simulink model "NavigationRocketPlant"  (R2025b)
settings: Solver=ode5  StartTime=0.0  StopTime=350  RelTol=1e-3
PostLoadFcn:
  | addpath('settings/')
  | addpath('settings/environment/')
  | 
  | run sensorSettings.m
InitFcn:
  | run(fullfile(fileparts(get_param(bdroot,'FileName')),'..','rocketPlantMain.m'))
undefined symbols (not defined in the file): Airbrake, AirbrakeInitialState, ba0, bg0, CdLookup, DiscIntNeverNeededParam, dspblkCoreblockFVToolHelper, Environment, gcbh, GNSSConfig, GNSSInitialState, LLA0, MEKF, p0, P0, pressure0, q0, Rocket, RocketInitialState, Sensor, stationaryTime, v0, Weather
libraries: simulink x2, dspmathops x1
(part 3 of 3)

== matlab function NavigationRocketPlant/Sensors/GNSS/GNSS_Receiver ==
  data: truth_NEU input; LLA_deg_m output; fix_info output; time_s input; reference input; state_in input Bus: GNSSReceiverStateBus; GNSSConfig parameter; state_out output Bus: GNSSReceiverStateBus
function [LLA_deg_m, fix_info, state_out] = GNSSReceiver( ...
    truth_NEU, time_s, reference, state_in, GNSSConfig)
% Position only: latitude [deg], longitude [deg], ellipsoid height [m].
% Acquisition error and metadata are delayed together; no velocity output.
% All noise streams, correlated errors and delayed packets are explicit.
% GNSS_State (Unit Delay) supplies the initialized state and stores updates.
state_out = state_in;
%GNSSPOSITIONSTEP Acquire, perturb and deliver a position-only GNSS fix.
%   truth_NEU = [north; east; absolute_altitude; vNorth; vEast; vUp], SI.
%   LLA_deg_m = [latitude_deg; longitude_deg; absolute_altitude_m]. The altitude
%   datum is inherited from the trajectory; no geoid correction is implied.
%   fix_info = [fresh; valid; acquisitionTime; age; sigmaN; sigmaE; sigmaD;
%           reasonCode]. Sigmas describe aggregate metric NED position noise.
%   reasonCode is a bit mask: 1 invalid truth, 2 startup/specified outage,
%   4 conservative receiver dynamics gate, 8 reacquisition, 16 packet loss,
%   32 stale. A received invalid-fix packet is fresh but invalid. A packet
%   loss notification is neither fresh nor valid, and never changes LLA.
%
%   Correlated residuals aggregate post-solution atmospheric/orbit/receiver
%   effects. Ground multipath and quality/outlier windows are configurable
%   scenarios, not satellite-geometry predictions. Velocity truth is used
%   only to check the receiver envelope; GNSS velocity is never produced.
%   Call gnssPositionInitialize to reset before each simulation.

    assert(isequal(size(truth_NEU), [6, 1]));
    assert(isfinite(time_s) && time_s >= 0.0);
    tolerance = 1.0e-9 * max(1.0, abs(time_s));
    assert(time_s >= state_out.previousStepTime - tolerance);
    state_out.previousStepTime = time_s;

    if time_s >= state_out.nextAcquisitionTime - tolerance
        % Receiver clock Ts/TransportSubsteps hits every acquisition epoch.
        % If a standalone caller skips ticks after a gap,
        % acquire the current truth once; do not invent historical fixes.
        state_out.nextAcquisitionTime = ...
            (floor((time_s + tolerance) / GNSSConfig.Ts) + 1.0) * GNSSConfig.Ts;
        [packetLLA, packetInfo, state_out] = acquirePosition( ...
            truth_NEU, time_s, reference, GNSSConfig, state_out);
        assert(state_out.queueCount < 32.0);
        tail = mod(state_out.queueHead + state_out.queueCount - 1.0, 32.0) + 1.0;
        state_out.queueLLA(:, tail) = packetLLA;
        state_out.queueInfo(:, tail) = packetInfo;
        state_out.queueDueTime(tail) = time_s + GNSSConfig.Delay;
        state_out.queueCount = state_out.queueCount + 1.0;
    end

    fresh = 0.0;
    % Fixed-size loop is compatible with generated MATLAB Function code.
    for packet = 1:32
        if state_out.queueCount <= 0.0
            break;
        end
        head = state_out.queueHead;
        if state_out.queueDueTime(head) > time_s + tolerance
            break;
        end
        arrived = state_out.queueInfo(:, head);
        if arrived(2) > 0.5
            state_out.heldLLA = state_out.queueLLA(:, head);
        end
        state_out.heldInfo = arrived;
        fresh = max(fresh, arrived(1));
        state_out.queueDueTime(head) = realmax;
        state_out.queueHead = mod(head, 32.0) + 1.0;
        state_out.queueCount = state_out.queueCount - 1.0;
    end

    LLA_deg_m = state_out.heldLLA;
    fix_info = state_out.heldInfo;
    fix_info(1) = fresh;
    fix_info(4) = max(0.0, time_s - fix_info(3));
    if fix_info(4) > GNSSConfig.MaxAge + tolerance
        fix_info(2) = 0.0;
        if mod(floor(fix_info(8) / 32.0), 2.0) == 0.0
            fix_info(8) = fix_info(8) + 32.0;
        end
    end
% Hold the delivered-packet marker across the asynchronous rate transfer.
% GNSS_Consume produces the single fresh pulse at the IMU polling tick.
fix_info(1) = state_out.heldInfo(1);
LLA_deg_m(3) = LLA_deg_m(3) + GNSSConfig.GeoidSeparation;
end

function [lla, info, state] = acquirePosition( ...
    truthNEU6, time_s, referenceLLArad, cfg, state)
    white = zeros(3, 1);
    phiSlow = exp(-cfg.Ts / cfg.Correlated.Tau);
    phiMultipath = exp(-cfg.Ts / cfg.Multipath.Tau);
    for axis = 1:3
        [normalWhite, state.rng(axis)] = normalDraw(state.rng(axis));
        [normalSlow, state.rng(axis + 3)] = ...
            normalDraw(state.rng(axis + 3));
        [normalMultipath, state.rng(axis + 6)] = ...
            normalDraw(state.rng(axis + 6));
        white(axis) = cfg.Noise.White.Position.Sigma(axis) * normalWhite;
        state.slowErrorNED(axis) = phiSlow * state.slowErrorNED(axis) + ...
            cfg.Correlated.Sigma(axis) * sqrt(1.0 - phiSlow^2) * normalSlow;
        state.multipathErrorNED(axis) = ...
            phiMultipath * state.multipathErrorNED(axis) + ...
            cfg.Multipath.Sigma(axis) * ...
            sqrt(1.0 - phiMultipath^2) * normalMultipath;
    end
    [packetDraw, state.rng(10)] = uniformDraw(state.rng(10));

    truthValid = all(isfinite(truthNEU6));
    reason = 0.0;
    altitude = referenceLLArad(3);
    acceleration = 0.0;
    speed = 0.0;
    if truthValid
        altitude = truthNEU6(3);
        speed = sqrt(sum(truthNEU6(4:6).^2));
        if state.previousTruthValid
            elapsed = time_s - state.previousAcquisitionTime;
            if elapsed > 0.0
                acceleration = sqrt(sum((truthNEU6(4:6) - ...
                    state.previousVelocityNEU).^2)) / elapsed;
            end
        end
        state.previousVelocityNEU = truthNEU6(4:6);
    else
        reason = reason + 1.0;
    end
    state.previousTruthValid = truthValid;
    state.previousAcquisitionTime = time_s;

    if time_s < cfg.StartupTime
        reason = reason + 2.0;
    else
        for window = 1:size(cfg.OutageWindows, 1)
            if time_s >= cfg.OutageWindows(window, 1) && ...
                    time_s < cfg.OutageWindows(window, 2)
                reason = reason + 2.0;
                break;
            end
        end
    end
    if truthValid && cfg.EnforceDynamicsLimits && ...
            (acceleration > cfg.MaxAcceleration || ...
             altitude > cfg.MaxAltitude || speed > cfg.MaxVelocity)
        reason = reason + 4.0;
    end
    % StartupTime already represents time to first fix; do not add a second
    % reacquisition interval solely because the receiver was starting up.
    startupOnly = reason == 2.0 && time_s < cfg.StartupTime;
    if reason > 0.0 && ~startupOnly
        state.reacquisitionUntil = time_s + cfg.Ts + cfg.ReacquisitionTime;
    elseif reason == 0.0 && time_s < state.reacquisitionUntil - 1.0e-9
        reason = 8.0;
    end

    quality = 1.0;
    for window = 1:size(cfg.QualityWindows, 1)
        if time_s >= cfg.QualityWindows(window, 1) && ...
                time_s < cfg.QualityWindows(window, 2)
            quality = max(quality, cfg.QualityWindows(window, 3));
        end
    end
    taper = exp(-max(0.0, altitude - referenceLLArad(3)) / ...
        cfg.Multipath.HeightScale);
    sigmaNED = quality * sqrt(cfg.Noise.White.Position.Sigma.^2 + ...
        cfg.Correlated.Sigma.^2 + (taper * cfg.Multipath.Sigma).^2);

    lla = state.heldLLA;
    if reason == 0.0
        errorNED = cfg.Position.Bias + quality * (white + ...
            state.slowErrorNED + taper * state.multipathErrorNED);
        for window = 1:size(cfg.OutlierWindows, 1)
            if time_s >= cfg.OutlierWindows(window, 1) && ...
                    time_s < cfg.OutlierWindows(window, 2)
                errorNED = errorNED + cfg.OutlierWindows(window, 3:5)';
            end
        end
        measuredNEU = truthNEU6(1:3) + ...
            [errorNED(1); errorNED(2); -errorNED(3)];
        lla = gnssNeuToLla(measuredNEU, referenceLLArad);
        for axis = 1:3
            quantum = cfg.Position.QuantLLA(axis);
            if quantum > 0.0
                lla(axis) = round(lla(axis) / quantum) * quantum;
            end
        end
    end
    fresh = 1.0;
    valid = double(reason == 0.0);
    if packetDraw < cfg.PacketLossProbability
        reason = reason + 16.0;
        fresh = 0.0;
        valid = 0.0;
    end
    info = [fresh; valid; time_s; 0.0; sigmaNED; reason];
end

function [normal, seed] = normalDraw(seed)
    [uniform1, seed] = uniformDraw(seed);
    [uniform2, seed] = uniformDraw(seed);
    normal = sqrt(-2.0 * log(uniform1)) * cos(2.0 * pi * uniform2);
end

function [uniform, seed] = uniformDraw(seed)
    % Integer arithmetic stays exact within IEEE double's 53-bit mantissa.
    seed = mod(16807.0 * seed, 2147483647.0);
    uniform = seed / 2147483647.0;
end

== matlab function NavigationRocketPlant/Navigation/GNSS_LLA_to_NED ==
  data: llaDegM input; positionNED output; reference input; GNSSConfig parameter
function positionNED = GNSSLLAtoNED(llaDegM, reference, GNSSConfig)
% GPS output uses ellipsoid height. Restore the source altitude datum before
% conversion to local Down; never add the launch altitude a second time.
llaSourceDatum = llaDegM;
llaSourceDatum(3) = llaSourceDatum(3) - GNSSConfig.GeoidSeparation;
%GNSSLLATONED Convert a GNSS LLA fix to the local navigation frame.
%   llaSourceDatum is [latitude_deg; longitude_deg; absolute_altitude_m], 3-by-1.
%   reference is [latitude_rad; longitude_rad; altitude_m], 3-by-1.
%   positionNED is [north_m; east_m; down_m], a 3-by-1 vector.
%
%   This is the inverse of the small-area WGS-84 curvature approximation
%   used by the Environment truth conversion. Longitude differences wrap
%   across the antimeridian. Down is reference altitude minus fix altitude.
%   The source altitude datum is unspecified; no geoid conversion is made.

    assert(isequal(size(llaSourceDatum), [3, 1]));
    assert(isequal(size(reference), [3, 1]));

    semimajorAxis_m = 6378137.0;
    eccentricitySquared = 6.69437999014e-3;
    latitude0_rad = reference(1);
    longitude0_rad = reference(2);
    altitude0_m = reference(3);
    cosLatitude0 = cos(latitude0_rad);

    % Longitude is undefined at a reference pole in this local mapping.
    assert(abs(cosLatitude0) > 1.0e-12);
    sinLatitude0 = sin(latitude0_rad);
    denominator = 1.0 - eccentricitySquared * sinLatitude0^2;
    primeVerticalRadius_m = semimajorAxis_m / sqrt(denominator);
    meridianRadius_m = semimajorAxis_m * (1.0 - eccentricitySquared) / ...
        denominator^(3.0 / 2.0);

    latitude_rad = llaSourceDatum(1) * (pi / 180.0);
    longitude_rad = llaSourceDatum(2) * (pi / 180.0);
    longitudeDifference_rad = mod(longitude_rad - longitude0_rad + pi, ...
        2.0 * pi) - pi;

    north_m = (latitude_rad - latitude0_rad) * ...
        (meridianRadius_m + altitude0_m);
    east_m = longitudeDifference_rad * ...
        ((primeVerticalRadius_m + altitude0_m) * cosLatitude0);
    down_m = altitude0_m - llaSourceDatum(3);

    positionNED = [north_m; east_m; down_m];
end

== matlab function NavigationRocketPlant/Sensors/GNSS/GNSS_Consume ==
  data: packet input; LLA_deg_m output; time_s input; last_epoch_in input; fix_info output; last_epoch_out output; skipped_epochs output; GNSSConfig parameter
function [LLA_deg_m, fix_info, last_epoch_out, skipped_epochs] = GNSSConsume( ...
    packet, time_s, last_epoch_in, GNSSConfig)
% Stateless receiver-buffer polling; epoch memory is an explicit Unit Delay.
last_epoch_out = last_epoch_in;
%GNSSPACKETREAD Poll an atomic GNSS packet at the navigation/IMU rate.
%   packet = [LLA(3); metadata(8)], with metadata(1) a HELD received-packet
%   marker. Output metadata(1) pulses once per newly observed received epoch.
%   Recompute age at the consumer tick, including rate-transfer waiting.
%   Explicit last_epoch_out feedback resets to -1. Faster acquisition uses the
%   latest packet; skipped_epochs counts acquisition epochs not observed.

    assert(isequal(size(packet), [11, 1]));
    assert(isfinite(time_s) && time_s >= 0.0);
    LLA_deg_m = packet(1:3);
    fix_info = packet(4:11);
    skipped_epochs = 0.0;
    tolerance = 1.0e-9 * max(1.0, abs(time_s));
    epoch = fix_info(3);
    received = fix_info(1) > 0.5;
    lossNotification = mod(floor(fix_info(8) / 16.0), 2.0) == 1.0;
    validTime = isfinite(epoch) && epoch >= 0.0 && ...
        epoch <= time_s + tolerance;
    newEpoch = validTime && (received || lossNotification) && ...
        epoch > last_epoch_out + tolerance;
    if newEpoch
        if last_epoch_out >= 0.0
            skipped_epochs = max(0.0, round((epoch-last_epoch_out)/GNSSConfig.Ts)-1.0);
        else
            skipped_epochs = max(0.0, round(epoch/GNSSConfig.Ts));
        end
        last_epoch_out = epoch;
    end
    fix_info(1) = double(newEpoch && received);
    if validTime
        fix_info(4) = max(0.0, time_s - epoch);
    else
        fix_info(4) = 0.0;
        fix_info(2) = 0.0;
    end
    if fix_info(4) > GNSSConfig.MaxAge + tolerance
        fix_info(2) = 0.0;
        if mod(floor(fix_info(8) / 32.0), 2.0) == 0.0
            fix_info(8) = fix_info(8) + 32.0;
        end
    end
end

== matlab function NavigationRocketPlant/Enviroment/Rocket_dynamics/Rocket_step ==
  settings: updateMethod=DISCRETE  sampleTime=Rocket.Ts
  data: x input double size=17; xNext output double size=17; t input double size=1; g input double size=1; gustNED input double size=3; cdCommand input double size=1; cdEnabled input double size=1; Rocket parameter; Weather parameter
function xNext = rocketStep(x,t,g,gustNED,cdCommand,cdEnabled,Rocket,Weather)
% Algorithm and numeric helpers are embedded in this MATLAB Function block.
%ROCKETPLANTSTEP Explicit-state RK4 rocket dynamics and deterministic events.
% Advances Rocket.Ts from time t; substeps do not exceed Rocket.MaxStep.
% Both Cd control inputs are explicit block inputs.
% Events are localized by linear crossing interpolation (within a substep).
% Phase: 0 pad, 1 launch rail, 2 free, 3 drogue, 4 main, 5 landed.
% No persistent variables, randomness, file input or hidden object state.
% Parachutes apply forces with finite inflation; velocity remains continuous
% at deployment. Ground impact is the only velocity reset.
% Match the Environment driver: sample once per Rocket.Ts, then hold during
% the RK4 substeps. Altitude-dependent weather is still evaluated locally.
% Both control inputs are sampled at this major time and held for all stages.
    [cdCommand,cdEnabled]=rocketPlantValidateCdControl(cdCommand,cdEnabled);
    xNext=x;
    initial=rocketPlantInitialize(Rocket);
    launchR=rocketPlantRotation(initial(7:10));
    rail=launchR(:,3);
    n=max(1,ceil(Rocket.Ts/max(Rocket.MaxStep,eps)));
    dt=Rocket.Ts/n;
    for step=1:n
        time=t+(step-1)*dt;
        if xNext(14)<0.5
            [thrust,mass]=rocketPlantProperties(time,Rocket);
            direction=launchR*(Rocket.ThrustDirection/max(norm(Rocket.ThrustDirection),eps));
            if time>=Rocket.IgnitionTime && thrust*dot(direction,rail)+mass*g*rail(3)>0
                xNext(14)=1;
            end
        end
        xNext=activateDeployments(xNext,time);
        before=xNext;
        k1=rocketPlantDerivative(before,time,g,Rocket,Weather,gustNED,cdCommand,cdEnabled);
        k2=rocketPlantDerivative(before+0.5*dt*k1,time+0.5*dt,g,Rocket,Weather,gustNED,cdCommand,cdEnabled);
        k3=rocketPlantDerivative(before+0.5*dt*k2,time+0.5*dt,g,Rocket,Weather,gustNED,cdCommand,cdEnabled);
        k4=rocketPlantDerivative(before+dt*k3,time+dt,g,Rocket,Weather,gustNED,cdCommand,cdEnabled);
        xNext=before+dt*(k1+2*k2+2*k3+k4)/6;
        xNext(7:10)=xNext(7:10)/max(norm(xNext(7:10)),eps);
        endTime=time+dt;
        if xNext(14)>0.5 && xNext(14)<1.5
            distance=max(0,dot(xNext(1:3),rail));
            alongSpeed=dot(xNext(4:6),rail);
            if distance<=0
                alongSpeed=max(0,alongSpeed);
            end
            xNext(1:3)=rail*distance;
            xNext(4:6)=rail*alongSpeed;
            xNext(7:10)=initial(7:10);
            xNext(11:13)=zeros(3,1);
            if distance>=Rocket.RailLength
                xNext(14)=2;
            end
        end
        if xNext(14)>1.5 && xNext(14)<4.5
            % Record apogee when vertical NED velocity first crosses zero.
            if xNext(15)<0 && before(6)<0 && xNext(6)>=0
                fraction=max(0,min(1,-before(6)/max(xNext(6)-before(6),eps)));
                xNext(15)=time+fraction*dt;
                xNext(16)=xNext(15)+Rocket.DrogueLag;
            end
            % Main threshold only while descending, with independent latency.
            if xNext(15)>=0 && xNext(17)<0 && xNext(6)>0 && -xNext(3)<=Rocket.MainAltitudeAGL
                fraction=1;
                if -before(3)>Rocket.MainAltitudeAGL
                    fraction=max(0,min(1,(-before(3)-Rocket.MainAltitudeAGL)/ ...
                        max(xNext(3)-before(3),eps)));
                end
                xNext(17)=time+fraction*dt+Rocket.MainLag;
            end
            xNext=activateDeployments(xNext,endTime);
            % Plane ground contact; retain horizontal impact point and attitude.
            if xNext(3)>=0 && xNext(6)>0
                fraction=max(0,min(1,-before(3)/max(xNext(3)-before(3),eps)));
                xNext(1:2)=before(1:2)+fraction*(xNext(1:2)-before(1:2));
                xNext(3)=0;
                xNext(4:6)=zeros(3,1);
                xNext(11:13)=zeros(3,1);
                xNext(14)=5;
            end
        end
    end
    end
    
    function state=activateDeployments(state,time)
    if state(14)>1.5 && state(14)<4.5
        if state(17)>=0 && time>=state(17)
            state(14)=4;
        elseif state(16)>=0 && time>=state(16)
            state(14)=3;
        end
    end
end

function dx = rocketPlantDerivative(x,t,g,Rocket,Weather,gustNED,cdCommand,cdOverrideEnabled)
%ROCKETPLANTDERIVATIVE Continuous states; hybrid event states have zero rate.
% Local NED translation, body rates, active Hamilton scalar-last attitude.
    if nargin<5, Weather=[]; end
    if nargin<6, gustNED=rocketWeatherGust(t,Weather); end
    if nargin<7, cdCommand=0; end
    if nargin<8, cdOverrideEnabled=false; end
    [cdCommand,cdOverrideEnabled]=rocketPlantValidateCdControl(cdCommand,cdOverrideEnabled);
    dx=zeros(17,1);
    if x(14)<0.5 || x(14)>4.5
        return
    end
    [aN,alphaB]=rocketPlantLoads(x,t,g,Rocket,Weather,gustNED,cdCommand,cdOverrideEnabled);
    dx(1:3)=x(4:6);
    dx(4:6)=aN;
    q=x(7:10)/max(norm(x(7:10)),eps);
    w=x(11:13);
    dx(7:9)=0.5*(q(4)*w+cross(q(1:3),w));
    dx(10)=-0.5*dot(q(1:3),w);
    dx(11:13)=alphaB;
    if x(14)<1.5
        initial=rocketPlantInitialize(Rocket);
        launchR=rocketPlantRotation(initial(7:10));
        rail=launchR(:,3);
        dx(1:3)=rail*dot(x(4:6),rail);
        dx(7:13)=zeros(7,1);
    end
end

== matlab function NavigationRocketPlant/Enviroment/Rocket_dynamics/Rocket_kinematics ==
  settings: updateMethod=DISCRETE  sampleTime=Rocket.Ts
  data: x input double size=17; q output double size=4; w output double size=3; pNEU output double size=3; vNEU output double size=3; Rocket parameter; Weather parameter
function [q,w,pNEU,vNEU] = fcn(x,Rocket,Weather)
%#codegen
% Algorithm and numeric helpers are embedded in this MATLAB Function block.
%ROCKETPLANTKINEMATICS Existing Environment truth interface.
% Quaternion is body->NED xyzw. Position is [North;East;absolute MSL Up],
% velocity [North;East;Up]. Ellipsoid conversion remains in GNSS model.
q=x(7:10)/max(norm(x(7:10)),eps);
w=x(11:13);
pNEU=[x(1);x(2);Rocket.AltitudeMSL-x(3)];
vNEU=[x(4);x(5);-x(6)];
end

== matlab function NavigationRocketPlant/Enviroment/Rocket_dynamics/Rocket_force_truth ==
  settings: updateMethod=DISCRETE  sampleTime=Rocket.Ts
  data: x input double size=17; fB output double size=3; t input double size=1; g input double size=1; BNED input double size=3; gustNED input double size=3; cdCommand input double size=1; cdEnabled input double size=1; BB output double size=3; debug output double size=18; cdInfo output double size=5; Rocket parameter; Weather parameter
function [fB,BB,debug,cdInfo] = rocketForces(x,t,g,BNED,gustNED,cdCommand,cdEnabled,Rocket,Weather)
% Algorithm and numeric helpers are embedded in this MATLAB Function block.
%ROCKETPLANTFORCES Physical IMU specific force and body magnetic field.
% Includes rail/pad/ground support and acceleration at a rigid-body IMU
% offset. IMUOffset is measured from the lumped CM in body axes [m].
% debug is the fixed 18-vector documented in rocketPlantLoads.
% Cd command/enable use the same body drag as the state integrator.
% cdInfo is the separate five-element control diagnostic from rocketPlantLoads.
    [aN,alphaB,debug,cdInfo]=rocketPlantLoads(x,t,g,Rocket,Weather,gustNED,cdCommand,cdEnabled);
    R=rocketPlantRotation(x(7:10));
    w=x(11:13);
    r=Rocket.IMUOffset;
    fB=R.'*(aN-[0;0;g])+cross(alphaB,r)+cross(w,cross(w,r));
    BB=R.'*BNED;
end

== matlab function NavigationRocketPlant/Enviroment/Weather_conditions/Weather_truth ==
  settings: updateMethod=DISCRETE  sampleTime=Rocket.Ts
  data: positionNEU input double size=3; windNED output double size=3; t input double size=1; atmosphere output double size=5; gustNED output double size=3; Rocket parameter; Weather parameter
function [windNED,atmosphere,gustNED]= weatherFunction(positionNEU,t,Rocket,Weather)

% Complete atmosphere, mean-wind and explicit-time gust implementation.
% All runtime helpers are defined locally in this MATLAB Function block.
    gustNED=rocketWeatherGust(t,Weather);
    [windNED,rho,pressure,soundSpeed,temperature,RH]= ...
        rocketWeatherConditions(positionNEU(3),Rocket,Weather,gustNED);
    atmosphere=[rho;pressure;soundSpeed;temperature;RH];
end

== matlab function NavigationRocketPlant/Navigation/State Estimation/MEKF ==
  settings: updateMethod=DISCRETE  sampleTime=Sensor.Ts
  data: dt input; q_nb_out output; gyro_b input; acc_b input; baro_pressure_Pa input; mag_b input; h0_m input; gps_pos_n input; gps_fix_info input; mag_ref_n input; q_nb_in input; v_n_in input; p_n_in input; bg_in input; ba_in input; P_in input; use_acc_tilt input; mag_valid input; baro_valid input; gps_valid input; gps_frequency_Hz input; gps_timer_in input; v_n_out output; p_n_out output; bg_out output; ba_out output; P_out output; estimate_bias input; zeroUpdate input; gps_timer_out output; MEKF parameter; gps_diagnostic_out output; baro_calibration_out output double size=[2 1]; baro_calibration_in input double size=[2 1]; GNSSConfig parameter
function [q_nb_out, v_n_out, p_n_out, bg_out, ba_out, P_out, gps_timer_out, gps_diagnostic_out, baro_calibration_out] = MEKF_Navigation( ...
    dt, gyro_b, acc_b, baro_pressure_Pa, mag_b, h0_m, ...
    gps_pos_n, gps_fix_info, mag_ref_n, ...
    q_nb_in, v_n_in, p_n_in, bg_in, ba_in, P_in, ...
    use_acc_tilt, mag_valid, baro_valid, gps_valid, ...
    gps_frequency_Hz, gps_timer_in, ...
    estimate_bias, zeroUpdate, MEKF, baro_calibration_in, GNSSConfig)

    % -------------------------------------------------------------------------
    % Multiplicative Extended Kalman Filter for Navigation
    %
    % Sensors:
    %   gyro_b            : 3-axis gyroscope [rad/s]
    %   acc_b             : 3-axis accelerometer [m/s^2]
    %   mag_b             : 3-axis magnetometer [arbitrary unit or tesla]
    %   baro_pressure_Pa  : barometer pressure [Pa]
    %   gps_pos_n         : optional GPS position in local NED [m]
    %   gps_fix_info      : fresh/valid/acquisition time/age/NED sigma/status
    %   gps_frequency_Hz  : GPS update frequency [Hz]
    %   gps_timer_in      : last processed acquisition timestamp [s]
    %
    % Frame:
    %   n : local NED navigation frame
    %   b : body frame
    %
    % Quaternion:
    %   q_nb = [qx; qy; qz; qw], scalar-last
    %   q_nb maps body-frame vectors into navigation-frame vectors
    %
    % Nominal state:
    %   q_nb : attitude quaternion
    %   v_n  : velocity in NED [m/s]
    %   p_n  : position in NED [m]
    %   bg   : gyro bias [rad/s]
    %   ba   : accelerometer bias [m/s^2]
    %
    % Error state:
    %   dx = [dtheta; dv; dp; dbg; dba] in R^15
    %
    % Local NED convention:
    %   p_n(3) = D
    %   source-datum absolute altitude = h0_m - D
    %
    % -------------------------------------------------------------------------
    
    % -------------------------------------------------------------------------
    % Constants
    % -------------------------------------------------------------------------
    
    g0 = 9.80665;        % gravity magnitude [m/s^2]
    
    % -------------------------------------------------------------------------
    % Process diffusion tuning: Qd = G*Qc*G'*dt
    % -------------------------------------------------------------------------
    
    sigma_g = MEKF.sigma_g;
    sigma_a = MEKF.sigma_a;
    sigma_bg = MEKF.sigma_bg;
    sigma_ba = MEKF.sigma_ba;
    
    % -------------------------------------------------------------------------
    % Measurement-noise tuning
    % -------------------------------------------------------------------------
    
    sigma_acc_tilt = MEKF.sigma_acc_tilt;
    sigma_mag = MEKF.sigma_mag;
    sigma_baro_p = MEKF.sigma_baro_p;
    
    % Accelerometer update gate.
    % Accelerometer is used as gravity direction only when norm is close to g.
    acc_gate = MEKF.acc_gate;
    
    % -------------------------------------------------------------------------
    % Input protection
    % -------------------------------------------------------------------------
    
    if dt <= 0.0
        dt = 1.0e-3;
    end

    % -------------------------------------------------------------------------
    % GNSS delivery and duplicate/stale protection
    % -------------------------------------------------------------------------
    % A held receiver position is not a fresh measurement. Use the delivered
    % packet flags and timestamp, rather than a second independent 10 Hz timer.
    % Initialize the last processed timestamp to -1 so epoch zero is accepted.
    gps_timer = gps_timer_in;
    gps_update = 0;
    gps_age = gps_fix_info(4);
    gps_diagnostic = [0.0; 0.0; 0.0; gps_age];
    if gps_valid && gps_frequency_Hz > 0.0 && ...
            gps_fix_info(1) > 0.5 && gps_fix_info(2) > 0.5 && ...
            all(isfinite(gps_fix_info)) && gps_age >= 0.0 && ...
            gps_age <= GNSSConfig.MaxAge && ...
            gps_fix_info(3) > gps_timer_in + 1.0e-9 && ...
            all(gps_fix_info(5:7) >= 0.0)
        gps_update = 1;
        gps_timer = gps_fix_info(3);
        gps_diagnostic(1) = 1.0;
    end
    
    q_nb = quatNormalize(q_nb_in);
    v_n  = v_n_in;
    p_n  = p_n_in;
    bg   = bg_in;
    ba   = ba_in;
    

    P = 0.5 * (P_in + P_in');
    % Startup pressure zeroing at the known local origin.
    % Explicit Unit Delay state [offset_Pa; sample_count], initially [0;0].
    % Reset each simulation; freeze at launch. No sensor truth is used.
    baro_offset_Pa = baro_calibration_in(1);
    baro_samples = baro_calibration_in(2);
    if MEKF.baro_zero_enabled && zeroUpdate && baro_valid && isfinite(baro_pressure_Pa)
        [p_origin, ~] = ISA_model(0.0, h0_m);
        baro_samples = baro_samples + 1.0;
        baro_offset_Pa = baro_offset_Pa + ...
            (baro_pressure_Pa - p_origin - baro_offset_Pa) / baro_samples;
    end
    baro_pressure_calibrated = baro_pressure_Pa;
    if MEKF.baro_zero_enabled
        baro_pressure_calibrated = baro_pressure_Pa - baro_offset_Pa;
    end
    baro_calibration_out = [baro_offset_Pa; baro_samples];

    
    % -------------------------------------------------------------------------
    % Prediction step
    % -------------------------------------------------------------------------
    
    omega_b = gyro_b - bg;
    f_b     = acc_b  - ba;
    
    % Quaternion propagation.
    dq = deltaQuat(omega_b * dt);
    q_nb = quatNormalize(quatMultiply(q_nb, dq));
    
    % Rotation matrix from body frame to navigation frame.
    C_nb = quatToDcm(q_nb);
    
    % Strapdown translational propagation.
    % In NED, gravity is positive in the Down direction.
    g_n = [0.0; 0.0; g0];
    
    a_n = C_nb * f_b + g_n;
    
    p_n = p_n + v_n * dt + 0.5 * a_n * dt * dt;
    v_n = v_n + a_n * dt;
    
    % -------------------------------------------------------------------------
    % Covariance prediction
    % -------------------------------------------------------------------------
    
    F = zeros(15,15);
    
    % Attitude error dynamics:
    % dtheta_dot = -skew(omega_b) dtheta - dbg
    F(1:3,1:3)   = -skew3(omega_b);
    F(1:3,10:12) = -eye(3);
    
    % Velocity error dynamics:
    % dv_dot = -C_nb skew(f_b) dtheta - C_nb dba
    F(4:6,1:3)   = -C_nb * skew3(f_b);
    F(4:6,13:15) = -C_nb;
    
    % Position error dynamics:
    % dp_dot = dv
    F(7:9,4:6) = eye(3);
    
    % Bias dynamics:
    %   bg_dot = n_bg
    %   ba_dot = n_ba
    
    Phi = eye(15) + F * dt;
    
    G = zeros(15,12);
    
    G(1:3,1:3)     = -eye(3);   % gyro noise
    G(4:6,4:6)     = -C_nb;     % accelerometer noise
    G(10:12,7:9)   = eye(3);    % gyro bias random walk
    G(13:15,10:12) = eye(3);    % accelerometer bias random walk
    
    Qc = zeros(12,12);
    
    Qc(1:3,1:3)     = sigma_g^2  * eye(3);
    Qc(4:6,4:6)     = sigma_a^2  * eye(3);
    Qc(7:9,7:9)     = sigma_bg^2 * eye(3);
    Qc(10:12,10:12) = sigma_ba^2 * eye(3);
    
    Qd = G * Qc * G' * dt;
    
    P = Phi * P * Phi' + Qd;
    P = 0.5 * (P + P');

    
    if zeroUpdate
    
        [q_nb, v_n, p_n, bg, ba, P] = ZeroUpdateKalmanFilter( ...
            gyro_b, acc_b, q_nb, v_n, p_n, bg, ba, P, g0, estimate_bias, MEKF);
    
        C_nb = quatToDcm(q_nb);
    
    end

    % -------------------------------------------------------------------------
    % Accelerometer attitude update
    % -------------------------------------------------------------------------
    % The accelerometer update is used only when the acceleration norm is close
    % to gravity. Otherwise, the accelerometer contains significant translational
    % acceleration and should not be treated as a gravity vector.
    
    % Use the corrected bias; do not reuse the pre-zero-update value.
    f_b = acc_b - ba;
    acc_norm = norm3(f_b);
    
    if use_acc_tilt && ~zeroUpdate && acc_norm > 1.0e-6
    
        if abs(acc_norm - g0) < acc_gate * g0
    
            y_acc = f_b / acc_norm;
    
            C_bn = C_nb';
    
            g_unit_n = [0.0; 0.0; 1.0];
    
            % At rest, accelerometer measures approximately -gravity direction.
            yhat_acc = -C_bn * g_unit_n;
    
            H_acc = zeros(3,15);
            H_acc(:,1:3) = skew3(yhat_acc);
    
            [q_nb, v_n, p_n, bg, ba, P] = updateVector3( ...
                y_acc, yhat_acc, H_acc, sigma_acc_tilt^2, ...
                q_nb, v_n, p_n, bg, ba, P, estimate_bias);
    
            C_nb = quatToDcm(q_nb);
        end
    end
    
    % -------------------------------------------------------------------------
    % Magnetometer attitude update
    % -------------------------------------------------------------------------
    % Magnetometer measurement model:
    %
    %   z_m    = normalized measured magnetic field in body frame
    %   zhat_m = C_bn * m_ref_n
    %
    % where m_ref_n is the reference magnetic field in the navigation frame.
    
    mag_norm = norm3(mag_b);
    mag_ref_norm = norm3(mag_ref_n);
    
    if mag_valid && mag_norm > 1.0e-6 && mag_ref_norm > 1.0e-6
    
        y_mag = mag_b / mag_norm;
        m_ref_n = mag_ref_n / mag_ref_norm;
    
        C_bn = C_nb';
    
        yhat_mag = C_bn * m_ref_n;
    
        H_mag = zeros(3,15);
        H_mag(:,1:3) = skew3(yhat_mag);
    
        [q_nb, v_n, p_n, bg, ba, P] = updateVector3( ...
            y_mag, yhat_mag, H_mag, sigma_mag^2, ...
            q_nb, v_n, p_n, bg, ba, P, estimate_bias);
    
        C_nb = quatToDcm(q_nb);
    end
    
    % -------------------------------------------------------------------------
    % Barometer EKF update
    % -------------------------------------------------------------------------
    % The barometer is treated as a pressure sensor.
    %
    % Nonlinear measurement model:
    %
    %   z_b    = p_baro
    %   zhat_b = p_ISA(D)
    %
    % where:
    %
    %   D = p_n(3)
    %   h = h0_m - D
    %
    % The measurement Jacobian is:
    %
    %   H_b = dp_ISA/dD
    %
    % Since the error state contains dp at indices 7:9, the Down-position
    % derivative enters column 9.
    
    if baro_valid && isfinite(baro_pressure_calibrated)
    
        [p_hat, dp_dD] = ISA_model(p_n(3), h0_m);
    
        H_baro = zeros(1,15);
        H_baro(1,9) = dp_dD;
    
        [q_nb, v_n, p_n, bg, ba, P] = updateScalar( ...
            baro_pressure_calibrated, p_hat, H_baro, sigma_baro_p^2, ...
            q_nb, v_n, p_n, bg, ba, P, estimate_bias);
    
        C_nb = quatToDcm(q_nb);
    end
    
    % -------------------------------------------------------------------------
    % Optional GPS update
    % -------------------------------------------------------------------------

    if gps_update && all(isfinite(gps_pos_n))

        z_gps = gps_pos_n;
        % Short-latency kinematic observation at the acquisition time.
        % Uses Navigation's own state, never GNSS velocity or trajectory truth.
        % This bounded approximation is not a fixed-lag replay filter.
        acceleration_now = C_nb * (acc_b - ba) + [0.0;0.0;g0];
        zhat_gps = p_n - v_n * gps_age + ...
            0.5 * acceleration_now * gps_age^2;
        H_gps = zeros(3,15);
        H_gps(:,1:3) = -0.5 * gps_age^2 * C_nb * skew3(acc_b - ba);
        H_gps(:,4:6) = -gps_age * eye(3);
        H_gps(:,7:9) = eye(3);
        H_gps(:,13:15) = -0.5 * gps_age^2 * C_nb;
        latency_sigma = 0.5 * GNSSConfig.Navigation.LatencyAccelerationSigma * gps_age^2;
        % Per-fix metric uncertainty includes white, slow and multipath terms.
        % Keep a finite numerical floor for deliberately noiseless test cases.
        R_gps = diag(max(gps_fix_info(5:7).^2 + latency_sigma^2,1.0e-8));
        residual_gps = z_gps - zhat_gps;
        innovation_covariance = H_gps * P * H_gps' + R_gps;
        gps_nis = residual_gps' * (innovation_covariance \ residual_gps);
        gps_diagnostic(3) = gps_nis;
        % Reject the entire GNSS correction for a large outlier. This differs
        % from the existing bias-learning gate, which only protects ba.
        if isfinite(gps_nis) && gps_nis <= GNSSConfig.Navigation.NISLimit
        gps_diagnostic(2) = 1.0;

        % Position residuals can observe accelerometer bias through the
        % propagated p-v-ba covariance. Do not use GPS velocity or truth.
        learn_acc_bias = estimate_bias || (MEKF.acc_bias_flight_enabled && ...
            ~zeroUpdate && all(isfinite(f_b)) && ...
            norm3(f_b) <= MEKF.acc_bias_force_max);
        if estimate_bias
            bias_step_limit = inf;
            bias_nis_limit = inf;
        else
            bias_step_limit = MEKF.acc_bias_max_rate * ...
                max(dt, 1.0 / gps_frequency_Hz);
            bias_nis_limit = MEKF.acc_bias_nis_max;
        end

        [q_nb, v_n, p_n, bg, ba, P] = updateVector3( ...
            z_gps, zhat_gps, H_gps, R_gps, ...
            q_nb, v_n, p_n, bg, ba, P, estimate_bias, ...
            learn_acc_bias, bias_step_limit, bias_nis_limit);
        if learn_acc_bias && ~estimate_bias
            % Uncalibrated gain/alignment errors are not random-walk bias.
            % Retain an uncertainty allowance instead of becoming overconfident.
            % Adding only a nonnegative diagonal preserves covariance PSD.
            for axis = 1:3
                index = 12 + axis;
                P(index,index) = max(P(index,index), ...
                    MEKF.acc_bias_variance_floor);
            end
        end
        C_nb = quatToDcm(q_nb);
        end
    end

    % Outputs
    % -------------------------------------------------------------------------
    
    q_nb_out = quatNormalize(q_nb);
    v_n_out  = v_n;
    p_n_out  = p_n;
    bg_out   = bg;
    ba_out   = ba;
    P_out    = 0.5 * (P + P');
    gps_timer_out = gps_timer;
    gps_diagnostic_out = gps_diagnostic; % [fresh valid request; accepted; NIS; age]
    
end


%% Zero Update Kalman Filter
function [q, v, p, bg, ba, P] = ZeroUpdateKalmanFilter(gyro_b, acc_b, q, v, p, bg, ba, P, g0, estimate_bias, MEKF)


    % -------------------------------------------------------------------------
    % Stationary zero-update Kalman correction for MEKF
    %
    % This block assumes:
    %   - the sensor is not translating
    %   - the sensor is not rotating
    %   - velocity should be zero
    %   - accelerometer measures only gravity plus bias
    %   - gyroscope measures only bias
    %
    % State error:
    %   dx = [dtheta; dv; dp; dbg; dba]
    % -------------------------------------------------------------------------
    
    % Tuning values.
    % Start conservative, then reduce after checking residuals.
    sigma_zupt_v = MEKF.sigma_zupt_v;
    sigma_zaru_g = MEKF.sigma_zaru_g;
    sigma_acc_b = MEKF.sigma_acc_b;
    sigma_zp_p = MEKF.sigma_zp_p;
    
    % -------------------------------------------------------------------------
    % 1) Zero-velocity update, ZUPT
    % -------------------------------------------------------------------------
    % Measurement:
    %   z_v = 0
    %   zhat_v = v
    %
    % Jacobian:
    %   H_v = [0 I 0 0 0]
    
    z_zupt = zeros(3,1);
    zhat_zupt = v;
    
    H_zupt = zeros(3,15);
    H_zupt(:,4:6) = eye(3);
    
    [q, v, p, bg, ba, P] = updateVector3( ...
        z_zupt, zhat_zupt, H_zupt, sigma_zupt_v^2, ...
        q, v, p, bg, ba, P, estimate_bias);
    
    % -------------------------------------------------------------------------
    % 2) Zero-angular-rate update, ZARU
    % -------------------------------------------------------------------------
    % Stationary gyroscope model:
    %   gyro_b = bg + noise
    %
    % Measurement:
    %   z_g = gyro_b
    %   zhat_g = bg
    %
    % Jacobian:
    %   H_g = [0 0 0 I 0]
    
    z_zaru = gyro_b;
    zhat_zaru = bg;
    
    H_zaru = zeros(3,15);
    H_zaru(:,10:12) = eye(3);
    
    [q, v, p, bg, ba, P] = updateVector3( ...
        z_zaru, zhat_zaru, H_zaru, sigma_zaru_g^2, ...
        q, v, p, bg, ba, P, estimate_bias);
    
    % -------------------------------------------------------------------------
    % 3) Stationary accelerometer-bias update
    % -------------------------------------------------------------------------
    % Stationary accelerometer model:
    %   acc_b = -C_bn*g_n + ba + noise
    %
    % This is the update that directly helps accelerometer-bias convergence.
    %
    % Measurement:
    %   z_a = acc_b
    %   zhat_a = -C_bn*g_n + ba
    %
    % Jacobian:
    %   H_a = [d(acc)/dtheta, 0, 0, 0, I]
    
    C_nb = quatToDcm(q);
    C_bn = C_nb';
    
    g_n = [0.0; 0.0; g0];
    
    f_grav_b = -C_bn * g_n;
    
    z_acc = acc_b;
    zhat_acc = f_grav_b + ba;
    
    H_acc = zeros(3,15);
    
    % Attitude sensitivity.
    % This sign is consistent with the attitude-error convention used in the
    % previous accelerometer and magnetometer updates.
    H_acc(:,1:3) = skew3(f_grav_b);
    
    % Direct accelerometer-bias sensitivity.
    H_acc(:,13:15) = eye(3);
    
    [q, v, p, bg, ba, P] = updateVector3( ...
        z_acc, zhat_acc, H_acc, sigma_acc_b^2, ...
        q, v, p, bg, ba, P, estimate_bias);
    
    % -------------------------------------------------------------------------
    % 4) Zero-Position update
    % -------------------------------------------------------------------------
    % Use this only if the sensor is fixed at the local origin during the stationary phase.

    z_zp = [0; 0; 0];
    zhat_zp = p;

    H_zp = zeros(3,15);
    H_zp(:,7:9) = eye(3);

    [q, v, p, bg, ba, P] = updateVector3( ...
        z_zp, zhat_zp, H_zp, sigma_zp_p^2, ...
        q, v, p, bg, ba, P, estimate_bias);

end

== matlab function NavigationRocketPlant/Navigation/NED to LLA ==
  data: p_N input; LLA output; LLA0 input
function LLA = NED2LLA(p_N, LLA0)

    % p_N  = [north; east; down] in meters
    % LLA0 = [lat0; lon0; h0]
    % lat0, lon0 in rad
    % h0 in m
    %
    % LLA output = [lat; lon; h]
    % lat, lon in rad
    % h in m
    
    % WGS-84 constants
    a = 6378137.0;
    e2 = 6.69437999014e-3;
    
    lat0 = LLA0(1);
    lon0 = LLA0(2);
    h0   = LLA0(3);
    
    north = p_N(1);
    east  = p_N(2);
    down = p_N(3);
    
    sinLat = sin(lat0);
    
    RN = a / sqrt(1 - e2*sinLat^2);
    RM = a*(1 - e2) / (1 - e2*sinLat^2)^(3/2);
    
    lat = lat0 + north/(RM + h0);
    lon = lon0 + east/((RN + h0)*cos(lat0));
    h   = h0 - down;
    
    LLA = [lat; lon; h];

end

== matlab function NavigationRocketPlant/Enviroment/System/MATLAB Function ==
  data: h input; p output
function p = ISA_altitude_to_pressure(h)

    % ISA altitude-to-pressure conversion for the troposphere.
    %
    % Input:
    %   h : altitude above sea level [m]
    %
    % Output:
    %   p : static pressure [Pa]
    %
    % Assumptions:
    %   - ISA troposphere model
    %   - sea-level pressure p0 = 101325 Pa
    %   - valid approximately for h < 11 km
    
    T0 = 288.15;       % sea-level standard temperature [K]
    L  = 0.0065;       % temperature lapse rate [K/m]
    R  = 287.05;       % specific gas constant for air [J/(kg K)]
    g0 = 9.80665;      % gravitational acceleration [m/s^2]
    p0 = 101325.0;     % sea-level standard pressure [Pa]
    
    exponent = g0 / (R * L);
    
    p = p0 * (1.0 - (L * h) / T0)^exponent;

end
